simulink model "pendubotSimulink"  (R2024b)
settings: Solver=FixedStepDiscrete  StartTime=0.0  StopTime=10  FixedStep=0.01  RelTol=1e-3
InitFcn:
  | simpb_init
undefined symbols (not defined in the file or in its folder): ctrb, dt, eqb, mvar, pvar, Q, q1dref, q1ref, q2dref, q2ref, R, rank, uref
libraries: sharedTrackingLibrary x1
settings Model: Creator=heeirthan  LastModifiedBy=heeirthan

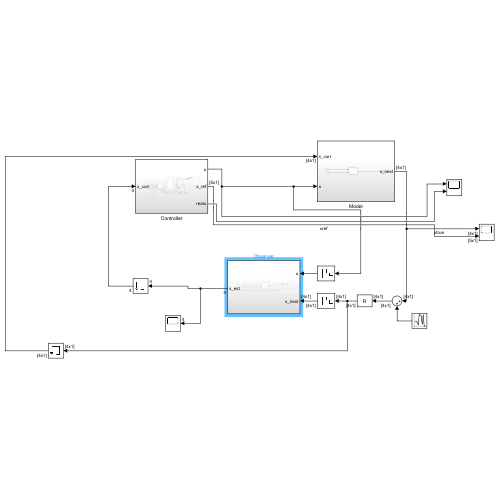
[thumbnail: Simulink's stored preview of the top-level diagram]
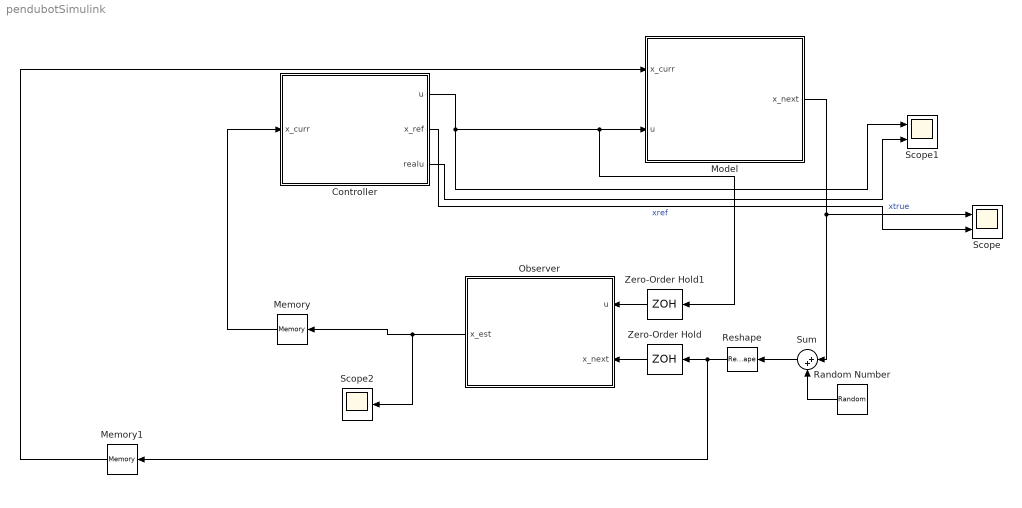
== system pendubotSimulink ==
  Controller : Subsystem
  Memory : Memory  InitialCondition=[-pi/2;0;0;0]
  Memory1 : Memory  InitialCondition=[-pi/2;0;0;0]
  Model : Subsystem
  Observer : Subsystem
  Random Number : RandomNumber  Variance=pvar  SampleTime=dt
  Reshape : Reshape  OutputDimensionality=Customize  OutputDimensions=[4,1]
  Scope : Scope  NumInputPorts=2
  Scope1 : Scope  NumInputPorts=2
  Scope2 : Scope
  Sum : Sum  Inputs=|++
  Zero-Order Hold : ZeroOrderHold  SampleTime=dt
  Zero-Order Hold1 : ZeroOrderHold  SampleTime=dt
  wires:
  Observer/1(x_est) -> Scope2/1, Memory/1
  Model/1(x_next) -> Sum/1, Scope/1  "xtrue"
  Controller/2(x_ref) -> Scope/2  "xref"
  Controller/3(realu) -> Scope1/2
  Controller/1(u) -> Zero-Order Hold1/1, Model/2(u), Scope1/1
  Memory/1 -> Controller/1(x_curr)
  Zero-Order Hold/1 -> Observer/2(x_next)
  Zero-Order Hold1/1 -> Observer/1(u)
  Sum/1 -> Reshape/1
  Reshape/1 -> Memory1/1, Zero-Order Hold/1
  Memory1/1 -> Model/1(x_curr)
  Random Number/1 -> Sum/2

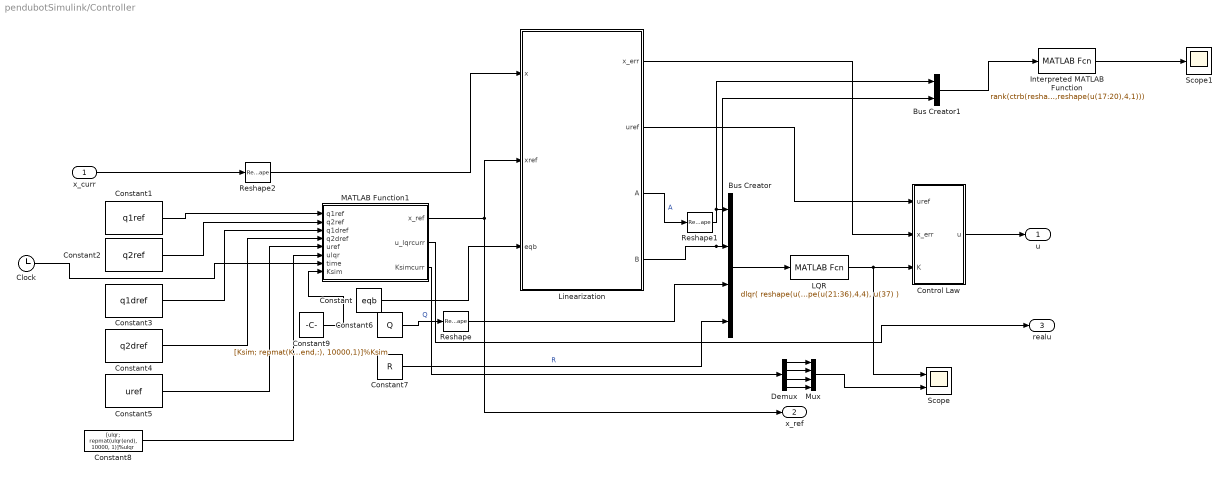
== system pendubotSimulink/Controller ==
  x_curr : Inport
  Bus Creator : BusCreator  Inputs=4
  Bus Creator1 : BusCreator  Inputs=2
  Clock : Clock
  Constant : Constant  Value=eqb
  Constant1 : Constant  Value=q1ref  SampleTime=-1
  Constant2 : Constant  Value=q2ref  SampleTime=-1
  Constant3 : Constant  Value=q1dref  SampleTime=-1
  Constant4 : Constant  Value=q2dref  SampleTime=-1
  Constant5 : Constant  Value=uref  SampleTime=-1
  Constant6 : Constant  Value=Q  SampleTime=-1
  Constant7 : Constant  Value=R  SampleTime=-1
  Constant8 : Constant  Value=[ulqr; repmat(ulqr(end), 10000, 1)]%ulqr  SampleTime=-1
  Constant9 : Constant  Value=[Ksim; repmat(Ksim(end,:), 10000,1)]%Ksim
  Control Law : MATLAB Function  TreatAsAtomicUnit=on
  Demux : Demux
  Interpreted MATLAB Function : MATLABFcn  MATLABFcn=rank(ctrb(reshape(u(1:16),4,4),reshape(u(17:20),4,1)))  Output1D=off
  LQR : MATLABFcn  MATLABFcn=dlqr( reshape(u(1:16),4,4), reshape(u(17:20),4,1), reshape(u(21:36),4,4), u(37) )  OutputDimensions=[1,4]  Output1D=off
  Linearization : MATLAB Function  TreatAsAtomicUnit=on
  MATLAB Function1 : MATLAB Function  TreatAsAtomicUnit=on
  Mux : Mux
  Reshape : Reshape
  Reshape1 : Reshape
  Reshape2 : Reshape  OutputDimensionality=Customize  OutputDimensions=[4,1]
  Scope : Scope  NumInputPorts=2
  Scope1 : Scope
  u : Outport
  x_ref : Outport  Port=2
  realu : Outport  Port=3
  wires:
  x_curr/1 -> Reshape2/1
  MATLAB Function1/1(x_ref) -> x_ref/1, Linearization/2(xref)
  Constant/1 -> Linearization/3(eqb)
  Linearization/3(A) -> Reshape1/1  "A"
  Linearization/4(B) -> Bus Creator1/2, Bus Creator/2
  Constant6/1 -> Reshape/1  "Q"
  Constant7/1 -> Bus Creator/4  "R"
  Bus Creator/1 -> LQR/1
  LQR/1 -> Scope/1, Control Law/3(K)
  Control Law/1(u) -> u/1
  Reshape/1 -> Bus Creator/3
  Reshape1/1 -> Bus Creator1/1, Bus Creator/1
  Linearization/2(uref) -> Control Law/1(uref)
  Linearization/1(x_err) -> Control Law/2(x_err)
  Reshape2/1 -> Linearization/1(x)
  Constant1/1 -> MATLAB Function1/1(q1ref)
  Constant2/1 -> MATLAB Function1/2(q2ref)
  Constant3/1 -> MATLAB Function1/3(q1dref)
  Constant4/1 -> MATLAB Function1/4(q2dref)
  Constant5/1 -> MATLAB Function1/5(uref)
  Constant8/1 -> MATLAB Function1/6(ulqr)
  MATLAB Function1/2(u_lqrcurr) -> realu/1
  Clock/1 -> MATLAB Function1/7(time)
  Constant9/1 -> MATLAB Function1/8(Ksim)
  Demux/1 -> Mux/1
  Demux/2 -> Mux/2
  Demux/3 -> Mux/3
  Demux/4 -> Mux/4
  Mux/1 -> Scope/2
  MATLAB Function1/3(Ksimcurr) -> Demux/1
  Bus Creator1/1 -> Interpreted MATLAB Function/1
  Interpreted MATLAB Function/1 -> Scope1/1

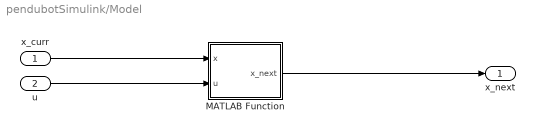
== system pendubotSimulink/Model ==
  x_curr : Inport
  u : Inport  Port=2
  MATLAB Function : MATLAB Function  TreatAsAtomicUnit=on
  x_next : Outport
  wires:
  u/1 -> MATLAB Function/2(u)
  x_curr/1 -> MATLAB Function/1(x)
  MATLAB Function/1(x_next) -> x_next/1

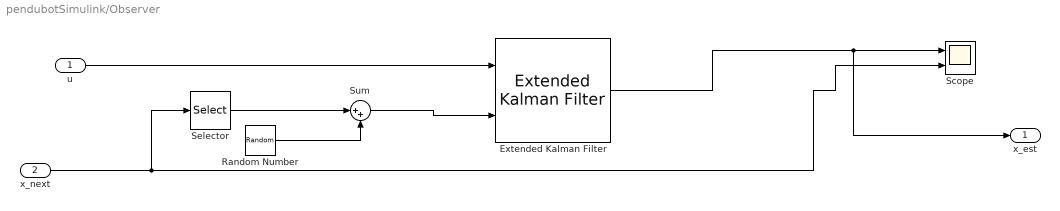
== system pendubotSimulink/Observer ==
  u : Inport
  x_next : Inport  Port=2
  Extended Kalman Filter : sharedTrackingLibrary/Extended Kalman Filter  StateTransitionFcn=EKF_stateFNpb  HasStateTransitionJacobianFcn=off  HasAdditiveProcessNoise=Additive  ProcessNoise=pNoise  HasTimeVaryingProcessNoise=off  HasStateTransitionFcnExtraArgument=1  InitialState=[-pi/2;0;0;0]  InitialStateCovariance=initvar  MeasurementFcn1=measurementFcn  HasMeasurementJacobianFcn1=off  HasMeasurementEnablePort1=off  HasAdditiveMeasurementNoise1=Additive  MeasurementNoise1=mNoise  HasTimeVaryingMeasurementNoise1=off  HasMeasurementFcnExtraArgument1=0  HasMeasurementWrapping1=off  MeasurementFcn2=myMeasurementFcn  HasMeasurementJacobianFcn2=off  HasMeasurementEnablePort2=off  HasAdditiveMeasurementNoise2=Additive  MeasurementNoise2=1  HasTimeVaryingMeasurementNoise2=off  HasMeasurementFcnExtraArgument2=0  HasMeasurementWrapping2=off  MeasurementFcn3=myMeasurementFcn  HasMeasurementJacobianFcn3=off  HasMeasurementEnablePort3=off  HasAdditiveMeasurementNoise3=Additive  MeasurementNoise3=1  HasTimeVaryingMeasurementNoise3=off  HasMeasurementFcnExtraArgument3=0  HasMeasurementWrapping3=off  MeasurementFcn4=myMeasurementFcn  HasMeasurementJacobianFcn4=off  HasMeasurementEnablePort4=off  HasAdditiveMeasurementNoise4=Additive  MeasurementNoise4=1  HasTimeVaryingMeasurementNoise4=off  HasMeasurementFcnExtraArgument4=0  HasMeasurementWrapping4=off  MeasurementFcn5=myMeasurementFcn  HasMeasurementJacobianFcn5=off  HasMeasurementEnablePort5=off  HasAdditiveMeasurementNoise5=Additive  MeasurementNoise5=1  HasTimeVaryingMeasurementNoise5=off  HasMeasurementFcnExtraArgument5=0  HasMeasurementWrapping5=off  EnableMultirate=off  StateTransitionFcnSampleTime=1  MeasurementFcn1SampleTime=1  MeasurementFcn2SampleTime=1  MeasurementFcn3SampleTime=1  MeasurementFcn4SampleTime=1  MeasurementFcn5SampleTime=1  UseCurrentEstimator=on  OutputStateCovariance=off  DataType=double  SampleTime=dt  NumberOfMeasurements=1
  Random Number : RandomNumber  Variance=mvar  SampleTime=dt
  Scope : Scope  NumInputPorts=2
  Selector : Selector  InputPortWidth=4  IndexOptions=Index vector (dialog)  Indices=[1 2]  OutputSizes=1
  Sum : Sum  Inputs=|++
  x_est : Outport
  wires:
  x_next/1 -> Scope/2, Selector/1
  u/1 -> Extended Kalman Filter/1
  Selector/1 -> Sum/1
  Sum/1 -> Extended Kalman Filter/2
  Random Number/1 -> Sum/2
  Extended Kalman Filter/1 -> x_est/1, Scope/1

== matlab function pendubotSimulink/Model/MATLAB Function ==
  data: x input; u input; x_next output; p parameter
function x_next = fcn(x, u, p)

dt = 0.01;
x_next = rk4_step(@(xx, uu) dx_pb_lqr(0,xx, uu, p), x, u,dt);
x_next(1) = wrapToPi(x_next(1));
x_next(2) = wrapToPi(x_next(2));
end

== matlab function pendubotSimulink/Controller/Linearization ==
  data: x_err output; uref output; x input; A output; xref input; eqb input; B output
function [x_err, uref, A,B]  = fcn(x,xref, eqb)

dt = 0.01;

q1ref = xref(1);
q2ref = xref(2);
q1dref = xref(3);
q2dref = xref(4);
uref = xref(5);


%Linearize about ref/equilibrium
if (norm([x(1);x(2)]-[pi/2;0]) > 0.6)
    %Linearize about current ref traj
    A = Afunfile(q1ref, q2ref, q1dref, q2dref, uref);
    B = Bfunfile(q1ref, q2ref, q1dref, q2dref, uref);
    
    x_err = [wrapToPi(x(1)-q1ref);
    wrapToPi(x(2)-q2ref);
    x(3) - q1dref;
    x(4)-q2dref];
else
    disp('In second controller')
    
    A = Afunfile(eqb(1), eqb(2), eqb(3), eqb(4), 0);
    B = Bfunfile(eqb(1), eqb(2), eqb(3), eqb(4), 0);

    x_err = [wrapToPi(x(1)-eqb(1));
    wrapToPi(x(2)-eqb(2));
    x(3) - eqb(3);
    x(4)-eqb(4)];
end


% Euler discretize here
A = eye(4) + dt*A;
B = dt * B;

== matlab function pendubotSimulink/Controller/MATLAB Function1 ==
  data: x_ref output; q1ref input; q2ref input; q1dref input; q2dref input; uref input; ulqr input; u_lqrcurr output; time input; Ksim input; Ksimcurr output
function [x_ref,u_lqrcurr, Ksimcurr] = fcn(q1ref,q2ref,q1dref,q2dref, uref, ulqr, time,Ksim)
dt = 0.01;
persistent t;
if isempty(t)
    t = 1;
else 
    t = t+1;
end

t
if t > length(q1ref)
    x_ref = [pi/2;0;0;0;0];
else    
    x_ref = [q1ref(t);q2ref(t);q1dref(t);q2dref(t);uref(t)];
    
end
u_lqrcurr = ulqr(t); %not used, just for plotting
Ksimcurr = Ksim(t,:);

== matlab function pendubotSimulink/Controller/Control Law ==
  data: uref input; x_err input; K input; u output
function u = fcn(uref,x_err,K)
K_max = 100; 
K = max(-K_max, min(K,K_max));
u = uref - K * x_err;
u_max = 20;
u = max(-u_max, min(u,u_max));
